simulink model "cirrusSR22T_v65"  (R2023a)
settings: Solver=ode45  StartTime=0.0  StopTime=360  FixedStep=0.001  MaxStep=0.1  RelTol=1e-3  EnableMultiTasking=on
values from neighbouring files (symbols this model uses):
  Aero_RP = [-1.145  0.0 -0.53]*[-1 0 0;0 1 0;0 0 -1]    [sr22t_data.m]
  aileron_limits = [-0.35 0.35]    [sr22t_data.m]
  Bw = 25.99*0.3048    (= 7.921752)    [sr22t_data.m]
  CD_alpha = [-1.57    1.500 ... (first row only)    [sr22t_data.m]
  CD_beta = [-1.57    1.230 ... (first row only)    [sr22t_data.m]
  CD_elev = 0.01    [sr22t_data.m]
  CD_ind = 0.007    [sr22t_data.m]
  CD_mach = [0, 0 ... (first row only)    [sr22t_data.m]
  Cl_ail = 0.1    [sr22t_data.m]
  CL_alpha = [-0.20 -0.750 ... (first row only)    [sr22t_data.m]
  Cl_beta = -0.1    [sr22t_data.m]
  CL_elev = 0.15    [sr22t_data.m]
  Cl_p = -0.4    [sr22t_data.m]
  CL_q = 3.9 * 0    (= 0)    [sr22t_data.m]
  Cl_r = 0.15    [sr22t_data.m]
  Cl_rudder = 0.01    [sr22t_data.m]
  Cm_alpha = -0.8    [sr22t_data.m]
  Cm_alpha_dot = -7    [sr22t_data.m]
  Cm_elev = [0.0, -1.100 ... (first row only)    [sr22t_data.m]
  Cm_q = -15    [sr22t_data.m]
  Cn_ail = -0.01    [sr22t_data.m]
  Cn_beta = 0.12    [sr22t_data.m]
  Cn_r = -0.15    [sr22t_data.m]
  Cn_rudder = -0.15    [sr22t_data.m]
  Cw = 5.58*0.3048    (= 1.700784)    [sr22t_data.m]
  CY_beta = -1    [sr22t_data.m]
  CY_p = [0.0000  -0.075 ... (first row only)    [sr22t_data.m]
  CY_r = [0.0000   0.214 ... (first row only)    [sr22t_data.m]
  CY_rudder = 0.187    [sr22t_data.m]
  Den = tf_linsys1(3,2).Denominator{1,1}    [controller_h_hold.m]
  elevator_limits = [-0.35 0.35]    [sr22t_data.m]
  He = tf_linsys1(3,2).Numerator{1,1}    [controller_h_hold.m]
  Href = 0.05 * x0(3)    [controller_h_hold.m]
  Ht = tf_linsys1(3,4).Numerator{1,1}    [controller_h_hold.m]
  isTrimming = 0    [sr22t_data.m]
  Jxx = 897*1.3558179    (= 1216.1686563)    [sr22t_data.m]
  Jxz = 0    [sr22t_data.m]
  Jyy = 20699*1.3558179    (= 28064.0747121)    [sr22t_data.m]
  Jzz = 19876*1.3558179    (= 26948.2365804)    [sr22t_data.m]
  Kp = 6    [controller_h_hold.m]
  kp = 0.005    [controller_h_hold.m]
  Kq = 3    [controller_h_hold.m]
  M = 2348*0.45359237    (= 1065.03488476)    [sr22t_data.m]
  Qe = tf_linsys1(8,2).Numerator{1,1}    [controller_h_hold.m]
  Qt = tf_linsys1(8,4).Numerator{1,1}    [controller_h_hold.m]
  Rcg = [-1.25 0.00 -0.54]*[-1 0 0;0 1 0;0 0 -1]    [sr22t_data.m]
  Rengine = [-3.6 0.0 -0.09045]*[-1 0 0;0 1 0;0 0 -1]    [sr22t_data.m]
  rudder_limits = [-0.35 0.35]    [sr22t_data.m]
  Sw = 144.92*0.09290304    (= 13.4635085568)    [sr22t_data.m]
  tau = 30    [controller_h_hold.m]
  Thetae = tf_linsys1(11,2).Numerator{1,1}    [controller_h_hold.m]
  Thetat = tf_linsys1(11,4).Numerator{1,1}    [controller_h_hold.m]
  thrust_limits = [0 1]    [sr22t_data.m]
  Ti = 17.5    [controller_h_hold.m]
  Tmax = M*10    (= 10650.3488476)    [sr22t_data.m]
  u0 = [op_trim1.Inputs(1,1).u, op_trim1.Inputs(2,1).u, op_trim1.Inputs(3,1).u, op_trim1.Inputs(4,1).u].'    [controller_h_hold.m]    (also in sr22t_data.m = [0, -0.013822, 0, 0.11837].')
  Ue = tf_linsys1(4,2).Numerator{1,1}    [controller_h_hold.m]
  Ut = tf_linsys1(4,4).Numerator{1,1}    [controller_h_hold.m]
  We = tf_linsys1(6,2).Numerator{1,1}    [controller_h_hold.m]
  Wt = tf_linsys1(6,4).Numerator{1,1}    [controller_h_hold.m]
  x0 = zeros(12,1)    [controller_h_hold.m]    (also in sr22t_data.m)
(part 2 of 2)

== system cirrusSR22T_v65/Cirrus SR22T/Aerodinamica/Forcas Aerodinamicas/Coef. Forca Lateral ==
  alpha : Inport
  beta : Inport  Port=2
  p : Inport  Port=3
  VT : Inport  Port=4
  r : Inport  Port=5
  rudder : Inport  Port=6
  CY_beta : Gain  Gain=CY_beta
  CY_p : Lookup  InputValues=CY_p(:,1);  Table=CY_p(:,2);  LookUpMeth=Interpolation-Use End Values
  CY_r : Lookup  InputValues=CY_r(:,1);  Table=CY_r(:,2);  LookUpMeth=Interpolation-Use End Values
  Constant2 : Constant  Value=Bw
  Gain : Gain  Gain=CY_rudder  SaturateOnIntegerOverflow=on  OutDataTypeStr=Inherit: Same as input  ParamDataTypeStr=Inherit: Same as input
  Gain1 : Gain  Gain=2  SaturateOnIntegerOverflow=on  OutDataTypeStr=Inherit: Same as input  ParamDataTypeStr=Inherit: Same as input
  Gain2 : Gain  Gain=0  SaturateOnIntegerOverflow=on  OutDataTypeStr=Inherit: Same as input  ParamDataTypeStr=Inherit: Same as input
  Gain3 : Gain  Gain=0  SaturateOnIntegerOverflow=on  OutDataTypeStr=Inherit: Same as input  ParamDataTypeStr=Inherit: Same as input
  Gain4 : Gain  Gain=0  SaturateOnIntegerOverflow=on  OutDataTypeStr=Inherit: Same as input  ParamDataTypeStr=Inherit: Same as input
  Product1 : Product  Inputs=3  SaturateOnIntegerOverflow=on  OutDataTypeStr=Inherit: Same as first input
  Product2 : Product  Inputs=3  SaturateOnIntegerOverflow=on  OutDataTypeStr=Inherit: Same as first input
  Product3 : Product  Inputs=*/  SaturateOnIntegerOverflow=on  OutDataTypeStr=Inherit: Same as first input
  Sum : Sum  Inputs=++++  SaturateOnIntegerOverflow=on
  C_Y : Outport
  wires:
  alpha/1 -> CY_p/1, CY_r/1
  beta/1 -> CY_beta/1
  Sum/1 -> C_Y/1
  CY_beta/1 -> Sum/1
  Product1/1 -> Sum/2
  p/1 -> Product1/2
  VT/1 -> Gain1/1
  Gain1/1 -> Product3/2
  Constant2/1 -> Product3/1
  Product3/1 -> Product1/3, Product2/1
  Product2/1 -> Sum/3
  CY_r/1 -> Gain2/1
  r/1 -> Product2/3
  Gain/1 -> Gain4/1
  rudder/1 -> Gain/1
  Gain2/1 -> Product2/2
  CY_p/1 -> Gain3/1
  Gain3/1 -> Product1/1
  Gain4/1 -> Sum/4

== system cirrusSR22T_v65/Cirrus SR22T/Aerodinamica/Forcas Aerodinamicas/Coef. sustentacao ==
  alpha : Inport
  elevator : Inport  Port=2
  VT : Inport  Port=3
  q : Inport  Port=4
  CL_alpha : Lookup  InputValues=CL_alpha(:,1);  Table=CL_alpha(:,2);  LookUpMeth=Interpolation-Use End Values
  Constant : Constant  Value=0
  Constant2 : Constant  Value=Cw
  Gain1 : Gain  Gain=2  SaturateOnIntegerOverflow=on  OutDataTypeStr=Inherit: Same as input  ParamDataTypeStr=Inherit: Same as input
  Gain2 : Gain  Gain=CL_q  SaturateOnIntegerOverflow=on  OutDataTypeStr=Inherit: Same as input  ParamDataTypeStr=Inherit: Same as input
  Gain3 : Gain  Gain=CL_elev  SaturateOnIntegerOverflow=on  OutDataTypeStr=Inherit: Same as input  ParamDataTypeStr=Inherit: Same as input
  Product2 : Product  SaturateOnIntegerOverflow=on  OutDataTypeStr=Inherit: Same as first input
  Product3 : Product  Inputs=*/  SaturateOnIntegerOverflow=on  OutDataTypeStr=Inherit: Same as first input
  Product4 : Product  SaturateOnIntegerOverflow=on  OutDataTypeStr=Inherit: Same as first input
  Sum1 : Sum  Inputs=++++  SaturateOnIntegerOverflow=on
  C_L : Outport
  wires:
  alpha/1 -> CL_alpha/1
  CL_alpha/1 -> Sum1/1
  Sum1/1 -> C_L/1
  Constant/1 -> Product2/1
  VT/1 -> Gain1/1
  Gain1/1 -> Product3/2
  Constant2/1 -> Product3/1
  Product2/1 -> Sum1/2
  Product3/1 -> Product2/2, Product4/2
  Gain2/1 -> Product4/1
  Product4/1 -> Sum1/3
  q/1 -> Gain2/1
  elevator/1 -> Gain3/1
  Gain3/1 -> Sum1/4

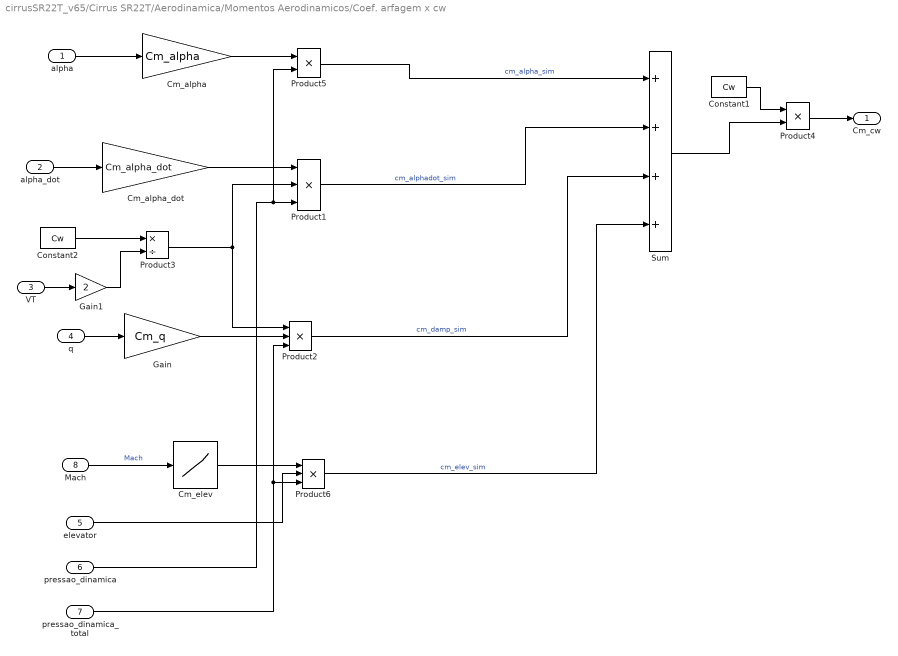
== system cirrusSR22T_v65/Cirrus SR22T/Aerodinamica/Momentos Aerodinamicos/Coef. arfagem x cw ==
  alpha : Inport
  alpha_dot : Inport  Port=2
  VT : Inport  Port=3
  q : Inport  Port=4
  elevator : Inport  Port=5
  pressao_dinamica : Inport  Port=6
  pressao_dinamica_total : Inport  Port=7
  Mach : Inport  Port=8
  Cm_alpha : Gain  Gain=Cm_alpha
  Cm_alpha_dot : Gain  Gain=Cm_alpha_dot
  Cm_elev : Lookup  InputValues=Cm_elev(:,1);  Table=Cm_elev(:,2);  LookUpMeth=Interpolation-Use End Values
  Constant1 : Constant  Value=Cw
  Constant2 : Constant  Value=Cw
  Gain : Gain  Gain=Cm_q  SaturateOnIntegerOverflow=on  OutDataTypeStr=Inherit: Same as input  ParamDataTypeStr=Inherit: Same as input
  Gain1 : Gain  Gain=2  SaturateOnIntegerOverflow=on  OutDataTypeStr=Inherit: Same as input  ParamDataTypeStr=Inherit: Same as input
  Product1 : Product  Inputs=***  SaturateOnIntegerOverflow=on  OutDataTypeStr=Inherit: Same as first input
  Product2 : Product  Inputs=***  SaturateOnIntegerOverflow=on  OutDataTypeStr=Inherit: Same as first input
  Product3 : Product  Inputs=*/  SaturateOnIntegerOverflow=on  OutDataTypeStr=Inherit: Same as first input
  Product4 : Product  Inputs=**  SaturateOnIntegerOverflow=on  OutDataTypeStr=Inherit: Same as first input
  Product5 : Product  Inputs=**  SaturateOnIntegerOverflow=on  OutDataTypeStr=Inherit: Same as first input
  Product6 : Product  Inputs=***  SaturateOnIntegerOverflow=on  OutDataTypeStr=Inherit: Same as first input
  Sum : Sum  Inputs=++++  SaturateOnIntegerOverflow=on
  Cm_cw : Outport
  wires:
  Constant1/1 -> Product4/1
  Sum/1 -> Product4/2
  Product4/1 -> Cm_cw/1
  VT/1 -> Gain1/1
  Gain1/1 -> Product3/2
  Constant2/1 -> Product3/1
  Cm_alpha_dot/1 -> Product1/1
  Product1/1 -> Sum/2  "cm_alphadot_sim"
  Product3/1 -> Product2/1, Product1/2
  q/1 -> Gain/1
  Gain/1 -> Product2/2
  Product2/1 -> Sum/3  "cm_damp_sim"
  elevator/1 -> Product6/2
  Mach/1 -> Cm_elev/1  "Mach"
  Cm_elev/1 -> Product6/1
  alpha_dot/1 -> Cm_alpha_dot/1
  alpha/1 -> Cm_alpha/1
  pressao_dinamica_total/1 -> Product2/3, Product6/3
  Product6/1 -> Sum/4  "cm_elev_sim"
  Cm_alpha/1 -> Product5/1
  Product5/1 -> Sum/1  "cm_alpha_sim"
  pressao_dinamica/1 -> Product5/2, Product1/3

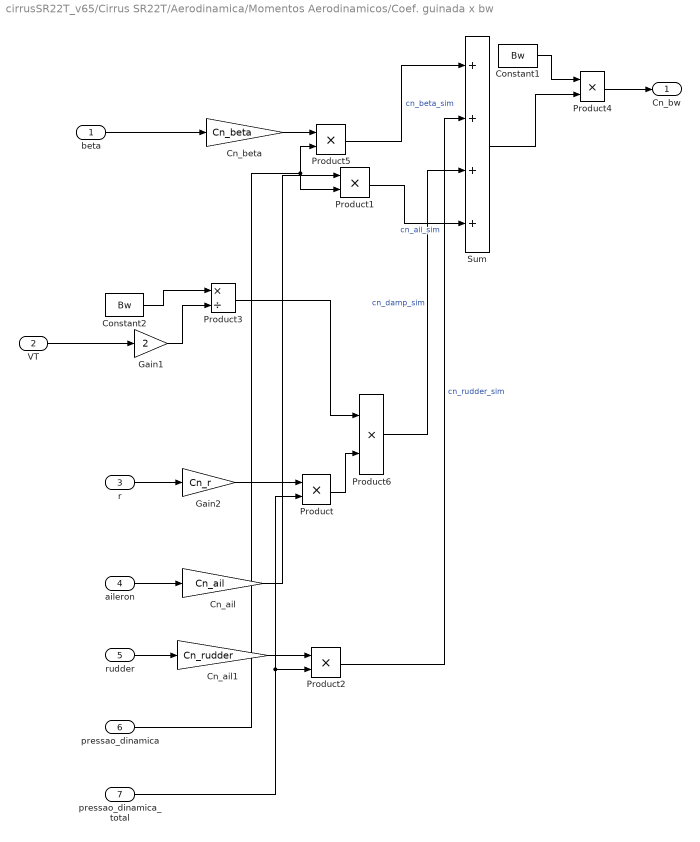
== system cirrusSR22T_v65/Cirrus SR22T/Aerodinamica/Momentos Aerodinamicos/Coef. guinada x bw ==
  beta : Inport
  VT : Inport  Port=2
  r : Inport  Port=3
  aileron : Inport  Port=4
  rudder : Inport  Port=5
  pressao_dinamica : Inport  Port=6
  pressao_dinamica_total : Inport  Port=7
  Cn_ail : Gain  Gain=Cn_ail  SaturateOnIntegerOverflow=on  OutDataTypeStr=Inherit: Same as input  ParamDataTypeStr=Inherit: Same as input
  Cn_ail1 : Gain  Gain=Cn_rudder  SaturateOnIntegerOverflow=on  OutDataTypeStr=Inherit: Same as input  ParamDataTypeStr=Inherit: Same as input
  Cn_beta : Gain  Gain=Cn_beta
  Constant1 : Constant  Value=Bw
  Constant2 : Constant  Value=Bw
  Gain1 : Gain  Gain=2  SaturateOnIntegerOverflow=on  OutDataTypeStr=Inherit: Same as input  ParamDataTypeStr=Inherit: Same as input
  Gain2 : Gain  Gain=Cn_r  SaturateOnIntegerOverflow=on  OutDataTypeStr=Inherit: Same as input  ParamDataTypeStr=Inherit: Same as input
  Product{,1..2,5} (4 alike) : Product
  Product3 : Product  Inputs=*/  SaturateOnIntegerOverflow=on  OutDataTypeStr=Inherit: Same as first input
  Product4 : Product  Inputs=**  SaturateOnIntegerOverflow=on  OutDataTypeStr=Inherit: Same as first input
  Product6 : Product  Inputs=**  SaturateOnIntegerOverflow=on  OutDataTypeStr=Inherit: Same as first input
  Sum : Sum  Inputs=++++  SaturateOnIntegerOverflow=on
  Cn_bw : Outport
  wires:
  Constant1/1 -> Product4/1
  Sum/1 -> Product4/2
  Product4/1 -> Cn_bw/1
  VT/1 -> Gain1/1
  Gain1/1 -> Product3/2
  Constant2/1 -> Product3/1
  beta/1 -> Cn_beta/1
  Product3/1 -> Product6/1
  r/1 -> Gain2/1
  Product6/1 -> Sum/3  "cn_damp_sim"
  aileron/1 -> Cn_ail/1
  rudder/1 -> Cn_ail1/1
  Gain2/1 -> Product/1
  Product/1 -> Product6/2
  pressao_dinamica_total/1 -> Product2/2, Product/2
  Cn_ail1/1 -> Product2/1
  Product2/1 -> Sum/2  "cn_rudder_sim"
  Cn_beta/1 -> Product5/1
  Product5/1 -> Sum/1  "cn_beta_sim"
  pressao_dinamica/1 -> Product1/2, Product5/2
  Product1/1 -> Sum/4  "cn_ail_sim"
  Cn_ail/1 -> Product1/1

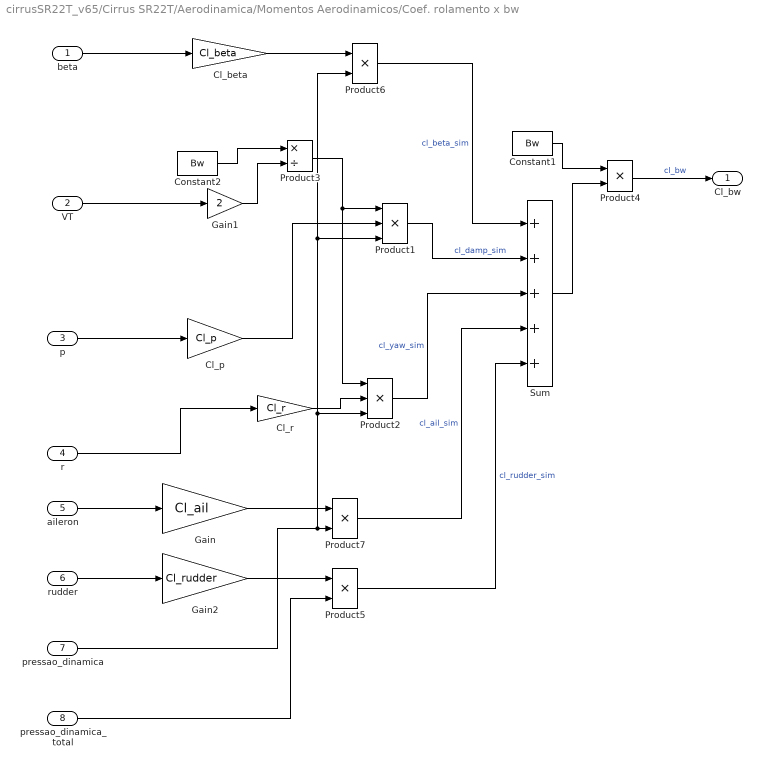
== system cirrusSR22T_v65/Cirrus SR22T/Aerodinamica/Momentos Aerodinamicos/Coef. rolamento x bw ==
  beta : Inport
  VT : Inport  Port=2
  p : Inport  Port=3
  r : Inport  Port=4
  aileron : Inport  Port=5
  rudder : Inport  Port=6
  pressao_dinamica : Inport  Port=7
  pressao_dinamica_total : Inport  Port=8
  Cl_beta : Gain  Gain=Cl_beta
  Cl_p : Gain  Gain=Cl_p
  Cl_r : Gain  Gain=Cl_r
  Constant1 : Constant  Value=Bw
  Constant2 : Constant  Value=Bw
  Gain : Gain  Gain=Cl_ail  SaturateOnIntegerOverflow=on  OutDataTypeStr=Inherit: Same as input  ParamDataTypeStr=Inherit: Same as input
  Gain1 : Gain  Gain=2  SaturateOnIntegerOverflow=on  OutDataTypeStr=Inherit: Same as input  ParamDataTypeStr=Inherit: Same as input
  Gain2 : Gain  Gain=Cl_rudder  SaturateOnIntegerOverflow=on  OutDataTypeStr=Inherit: Same as input  ParamDataTypeStr=Inherit: Same as input
  Product1 : Product  Inputs=3  SaturateOnIntegerOverflow=on  OutDataTypeStr=Inherit: Same as first input
  Product2 : Product  Inputs=3  SaturateOnIntegerOverflow=on  OutDataTypeStr=Inherit: Same as first input
  Product3 : Product  Inputs=*/  SaturateOnIntegerOverflow=on  OutDataTypeStr=Inherit: Same as first input
  Product4 : Product  Inputs=**  SaturateOnIntegerOverflow=on  OutDataTypeStr=Inherit: Same as first input
  Product5 : Product  SaturateOnIntegerOverflow=on  OutDataTypeStr=Inherit: Same as first input
  Product6 : Product  SaturateOnIntegerOverflow=on  OutDataTypeStr=Inherit: Same as first input
  Product7 : Product  SaturateOnIntegerOverflow=on  OutDataTypeStr=Inherit: Same as first input
  Sum : Sum  Inputs=+++++  SaturateOnIntegerOverflow=on
  Cl_bw : Outport
  wires:
  VT/1 -> Gain1/1
  Gain1/1 -> Product3/2
  Constant2/1 -> Product3/1
  Product3/1 -> Product2/1, Product1/1
  p/1 -> Cl_p/1
  r/1 -> Cl_r/1
  aileron/1 -> Gain/1
  rudder/1 -> Gain2/1
  Product1/1 -> Sum/2  "cl_damp_sim"
  Product2/1 -> Sum/3  "cl_yaw_sim"
  Constant1/1 -> Product4/1
  Sum/1 -> Product4/2
  Product4/1 -> Cl_bw/1  "cl_bw"
  beta/1 -> Cl_beta/1
  Cl_p/1 -> Product1/2
  Cl_r/1 -> Product2/2
  Gain2/1 -> Product5/1
  Product5/1 -> Sum/5  "cl_rudder_sim"
  pressao_dinamica_total/1 -> Product5/2
  pressao_dinamica/1 -> Product2/3, Product1/3, Product6/2, Product7/2
  Cl_beta/1 -> Product6/1
  Product6/1 -> Sum/1  "cl_beta_sim"
  Gain/1 -> Product7/1
  Product7/1 -> Sum/4  "cl_ail_sim"

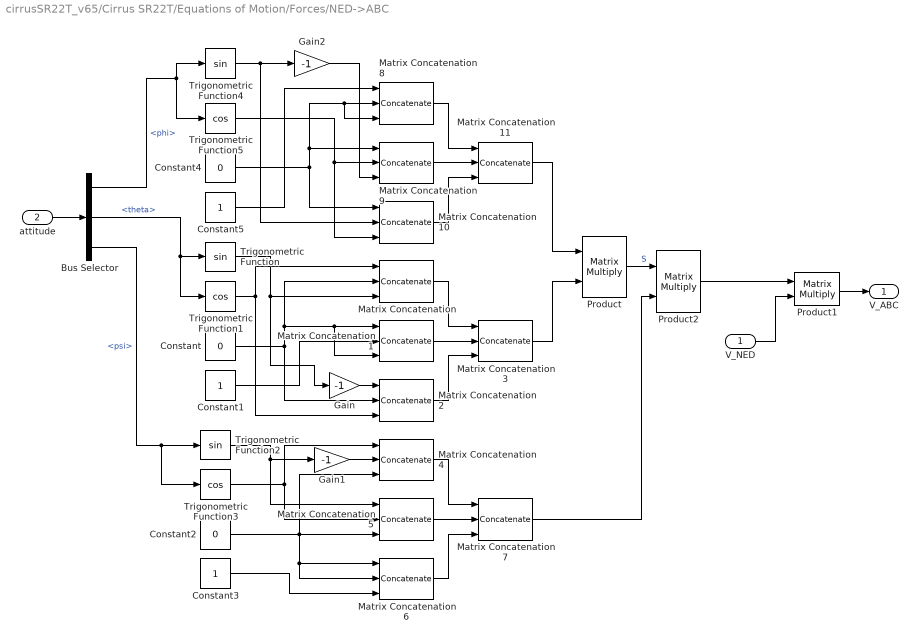
== system cirrusSR22T_v65/Cirrus SR22T/Equations of Motion/Forces/NED->ABC ==
  V_NED : Inport
  attitude : Inport  Port=2
  Bus Selector : BusSelector  OutputSignals=phi,theta,psi
  Constant : Constant  Value=0
  Constant1 : Constant
  Constant2 : Constant  Value=0
  Constant3 : Constant
  Constant4 : Constant  Value=0
  Constant5 : Constant
  Gain : Gain  Gain=-1  SaturateOnIntegerOverflow=on  OutDataTypeStr=Inherit: Same as input  ParamDataTypeStr=Inherit: Same as input
  Gain1 : Gain  Gain=-1  SaturateOnIntegerOverflow=on  OutDataTypeStr=Inherit: Same as input  ParamDataTypeStr=Inherit: Same as input
  Gain2 : Gain  Gain=-1  SaturateOnIntegerOverflow=on  OutDataTypeStr=Inherit: Same as input  ParamDataTypeStr=Inherit: Same as input
  Matrix Concatenation{,1..2,4..6,8..10} (9 alike) : Concatenate  NumInputs=3  Mode=Multidimensional array
  Matrix Concatenation11 : Concatenate  NumInputs=3  Mode=Multidimensional array  ConcatenateDimension=2
  Matrix Concatenation3 : Concatenate  NumInputs=3  Mode=Multidimensional array  ConcatenateDimension=2
  Matrix Concatenation7 : Concatenate  NumInputs=3  Mode=Multidimensional array  ConcatenateDimension=2
  Product : Product  Multiplication=Matrix(*)  SaturateOnIntegerOverflow=on  OutDataTypeStr=Inherit: Same as first input
  Product1 : Product  Multiplication=Matrix(*)  SaturateOnIntegerOverflow=on  OutDataTypeStr=Inherit: Same as first input
  Product2 : Product  Multiplication=Matrix(*)  SaturateOnIntegerOverflow=on  OutDataTypeStr=Inherit: Same as first input
  Trigonometric Function : Trigonometry
  Trigonometric Function1 : Trigonometry  Operator=cos
  Trigonometric Function2 : Trigonometry
  Trigonometric Function3 : Trigonometry  Operator=cos
  Trigonometric Function4 : Trigonometry
  Trigonometric Function5 : Trigonometry  Operator=cos
  V_ABC : Outport
  wires:
  Trigonometric Function1/1 -> Matrix Concatenation/1, Matrix Concatenation2/3
  Trigonometric Function/1 -> Matrix Concatenation/3, Gain/1
  Constant/1 -> Matrix Concatenation/2, Matrix Concatenation1/1, Matrix Concatenation1/3, Matrix Concatenation2/2
  Constant1/1 -> Matrix Concatenation1/2
  Matrix Concatenation/1 -> Matrix Concatenation3/1
  Matrix Concatenation1/1 -> Matrix Concatenation3/2
  Matrix Concatenation2/1 -> Matrix Concatenation3/3
  Matrix Concatenation4/1 -> Matrix Concatenation7/1
  Matrix Concatenation5/1 -> Matrix Concatenation7/2
  Matrix Concatenation6/1 -> Matrix Concatenation7/3
  Trigonometric Function3/1 -> Matrix Concatenation4/1, Matrix Concatenation5/2
  Trigonometric Function2/1 -> Gain1/1, Matrix Concatenation5/1
  Constant2/1 -> Matrix Concatenation4/3, Matrix Concatenation5/3, Matrix Concatenation6/1, Matrix Concatenation6/2
  Constant3/1 -> Matrix Concatenation6/3
  Product1/1 -> V_ABC/1
  attitude/1 -> Bus Selector/1
  Matrix Concatenation8/1 -> Matrix Concatenation11/1
  Matrix Concatenation9/1 -> Matrix Concatenation11/2
  Matrix Concatenation10/1 -> Matrix Concatenation11/3
  Bus Selector/1 -> Trigonometric Function4/1, Trigonometric Function5/1  "<phi>"
  Constant5/1 -> Matrix Concatenation8/1
  Constant4/1 -> Matrix Concatenation8/2, Matrix Concatenation8/3, Matrix Concatenation9/1, Matrix Concatenation10/1
  Trigonometric Function5/1 -> Matrix Concatenation9/2, Matrix Concatenation10/3
  Trigonometric Function4/1 -> Matrix Concatenation10/2, Gain2/1
  Bus Selector/2 -> Trigonometric Function/1, Trigonometric Function1/1  "<theta>"
  Bus Selector/3 -> Trigonometric Function2/1, Trigonometric Function3/1  "<psi>"
  Matrix Concatenation11/1 -> Product/1
  Matrix Concatenation3/1 -> Product/2
  V_NED/1 -> Product1/2
  Product/1 -> Product2/1  "S"
  Matrix Concatenation7/1 -> Product2/2
  Product2/1 -> Product1/1
  Gain2/1 -> Matrix Concatenation9/3
  Gain/1 -> Matrix Concatenation2/1
  Gain1/1 -> Matrix Concatenation4/2

== system cirrusSR22T_v65/Cirrus SR22T/Equations of Motion/Forces/Produto Vetorial ==
  V1 : Inport
  V2 : Inport  Port=2
  Mux : Mux  Inputs=2
  Mux1 : Mux  Inputs=3
  i : Fcn  Expr=u(2)*u(6)-u(3)*u(5)
  j : Fcn  Expr=-u(1)*u(6)+u(3)*u(4)
  k : Fcn  Expr=u(1)*u(5)-u(2)*u(4)
  V1 x V2 : Outport
  wires:
  V1/1 -> Mux/1
  V2/1 -> Mux/2
  Mux/1 -> i/1, j/1, k/1
  i/1 -> Mux1/1
  j/1 -> Mux1/2
  k/1 -> Mux1/3
  Mux1/1 -> V1 x V2/1

== system cirrusSR22T_v65/Cirrus SR22T/Equations of Motion/Forces/Produto Vetorial1 ==
  V1 : Inport
  V2 : Inport  Port=2
  Mux : Mux  Inputs=2
  Mux1 : Mux  Inputs=3
  i : Fcn  Expr=u(2)*u(6)-u(3)*u(5)
  j : Fcn  Expr=-u(1)*u(6)+u(3)*u(4)
  k : Fcn  Expr=u(1)*u(5)-u(2)*u(4)
  V1 x V2 : Outport
  wires:
  V1/1 -> Mux/1
  V2/1 -> Mux/2
  Mux/1 -> i/1, j/1, k/1
  i/1 -> Mux1/1
  j/1 -> Mux1/2
  k/1 -> Mux1/3
  Mux1/1 -> V1 x V2/1

== system cirrusSR22T_v65/Cirrus SR22T/Equations of Motion/Forces/Produto Vetorial2 ==
  V1 : Inport
  V2 : Inport  Port=2
  Mux : Mux  Inputs=2
  Mux1 : Mux  Inputs=3
  i : Fcn  Expr=u(2)*u(6)-u(3)*u(5)
  j : Fcn  Expr=-u(1)*u(6)+u(3)*u(4)
  k : Fcn  Expr=u(1)*u(5)-u(2)*u(4)
  V1 x V2 : Outport
  wires:
  V1/1 -> Mux/1
  V2/1 -> Mux/2
  Mux/1 -> i/1, j/1, k/1
  i/1 -> Mux1/1
  j/1 -> Mux1/2
  k/1 -> Mux1/3
  Mux1/1 -> V1 x V2/1

== system cirrusSR22T_v65/Cirrus SR22T/Equations of Motion/Forces/Produto Vetorial3 ==
  V1 : Inport
  V2 : Inport  Port=2
  Mux : Mux  Inputs=2
  Mux1 : Mux  Inputs=3
  i : Fcn  Expr=u(2)*u(6)-u(3)*u(5)
  j : Fcn  Expr=-u(1)*u(6)+u(3)*u(4)
  k : Fcn  Expr=u(1)*u(5)-u(2)*u(4)
  V1 x V2 : Outport
  wires:
  V1/1 -> Mux/1
  V2/1 -> Mux/2
  Mux/1 -> i/1, j/1, k/1
  i/1 -> Mux1/1
  j/1 -> Mux1/2
  k/1 -> Mux1/3
  Mux1/1 -> V1 x V2/1

== system cirrusSR22T_v65/Cirrus SR22T/Equations of Motion/Moments/Inertia ==
  Constant : Constant  Value=Jxx
  Constant1 : Constant  Value=Jyy
  Constant2 : Constant  Value=Jzz
  Constant3 : Constant  Value=-Jxz
  Constant4 : Constant  Value=0
  Matrix Concatenation10 : Concatenate  NumInputs=3  Mode=Multidimensional array
  Matrix Concatenation11 : Concatenate  NumInputs=3  Mode=Multidimensional array  ConcatenateDimension=2
  Matrix Concatenation8 : Concatenate  NumInputs=3  Mode=Multidimensional array
  Matrix Concatenation9 : Concatenate  NumInputs=3  Mode=Multidimensional array
  J : Outport
  wires:
  Matrix Concatenation8/1 -> Matrix Concatenation11/1
  Matrix Concatenation9/1 -> Matrix Concatenation11/2
  Matrix Concatenation10/1 -> Matrix Concatenation11/3
  Matrix Concatenation11/1 -> J/1
  Constant/1 -> Matrix Concatenation8/1
  Constant4/1 -> Matrix Concatenation8/2, Matrix Concatenation9/1, Matrix Concatenation9/3, Matrix Concatenation10/2
  Constant3/1 -> Matrix Concatenation8/3, Matrix Concatenation10/1
  Constant1/1 -> Matrix Concatenation9/2
  Constant2/1 -> Matrix Concatenation10/3

== system cirrusSR22T_v65/Cirrus SR22T/Equations of Motion/Moments/Inverse Inertia Matrix ==
  Constant : Constant  Value=Jzz
  Constant1 : Constant  Value=1/Jyy
  Constant2 : Constant  Value=Jxx
  Constant3 : Constant  Value=Jxz
  Constant4 : Constant  Value=0
  Constant5 : Constant  Value=Jxx*Jzz-Jxz^2
  Matrix Concatenation10 : Concatenate  NumInputs=3  Mode=Multidimensional array
  Matrix Concatenation11 : Concatenate  NumInputs=3  Mode=Multidimensional array  ConcatenateDimension=2
  Matrix Concatenation8 : Concatenate  NumInputs=3  Mode=Multidimensional array
  Matrix Concatenation9 : Concatenate  NumInputs=3  Mode=Multidimensional array
  Product : Product  Inputs=*/  SaturateOnIntegerOverflow=on  OutDataTypeStr=Inherit: Same as first input
  Product1 : Product  SaturateOnIntegerOverflow=on  OutDataTypeStr=Inherit: Same as first input
  inv J : Outport
  wires:
  Matrix Concatenation8/1 -> Matrix Concatenation11/1
  Matrix Concatenation9/1 -> Matrix Concatenation11/2
  Matrix Concatenation10/1 -> Matrix Concatenation11/3
  Constant/1 -> Matrix Concatenation8/1
  Constant4/1 -> Matrix Concatenation8/2, Matrix Concatenation9/1, Matrix Concatenation9/3, Matrix Concatenation10/2
  Constant3/1 -> Matrix Concatenation8/3, Matrix Concatenation10/1
  Constant2/1 -> Matrix Concatenation10/3
  Matrix Concatenation11/1 -> Product/1
  Product/1 -> inv J/1
  Constant5/1 -> Product/2, Product1/2
  Constant1/1 -> Product1/1
  Product1/1 -> Matrix Concatenation9/2

== system cirrusSR22T_v65/Cirrus SR22T/Equations of Motion/Moments/Produto Vetorial1 ==
  V1 : Inport
  V2 : Inport  Port=2
  Mux : Mux  Inputs=2
  Mux1 : Mux  Inputs=3
  i : Fcn  Expr=u(2)*u(6)-u(3)*u(5)
  j : Fcn  Expr=-u(1)*u(6)+u(3)*u(4)
  k : Fcn  Expr=u(1)*u(5)-u(2)*u(4)
  V1 x V2 : Outport
  wires:
  V1/1 -> Mux/1
  V2/1 -> Mux/2
  Mux/1 -> i/1, j/1, k/1
  i/1 -> Mux1/1
  j/1 -> Mux1/2
  k/1 -> Mux1/3
  Mux1/1 -> V1 x V2/1

== system cirrusSR22T_v65/Cirrus SR22T/Equations of Motion/Moments/Produto Vetorial2 ==
  V1 : Inport
  V2 : Inport  Port=2
  Mux : Mux  Inputs=2
  Mux1 : Mux  Inputs=3
  i : Fcn  Expr=u(2)*u(6)-u(3)*u(5)
  j : Fcn  Expr=-u(1)*u(6)+u(3)*u(4)
  k : Fcn  Expr=u(1)*u(5)-u(2)*u(4)
  V1 x V2 : Outport
  wires:
  V1/1 -> Mux/1
  V2/1 -> Mux/2
  Mux/1 -> i/1, j/1, k/1
  i/1 -> Mux1/1
  j/1 -> Mux1/2
  k/1 -> Mux1/3
  Mux1/1 -> V1 x V2/1

== system cirrusSR22T_v65/Cirrus SR22T/Equations of Motion/Moments/Produto Vetorial3 ==
  V1 : Inport
  V2 : Inport  Port=2
  Mux : Mux  Inputs=2
  Mux1 : Mux  Inputs=3
  i : Fcn  Expr=u(2)*u(6)-u(3)*u(5)
  j : Fcn  Expr=-u(1)*u(6)+u(3)*u(4)
  k : Fcn  Expr=u(1)*u(5)-u(2)*u(4)
  V1 x V2 : Outport
  wires:
  V1/1 -> Mux/1
  V2/1 -> Mux/2
  Mux/1 -> i/1, j/1, k/1
  i/1 -> Mux1/1
  j/1 -> Mux1/2
  k/1 -> Mux1/3
  Mux1/1 -> V1 x V2/1

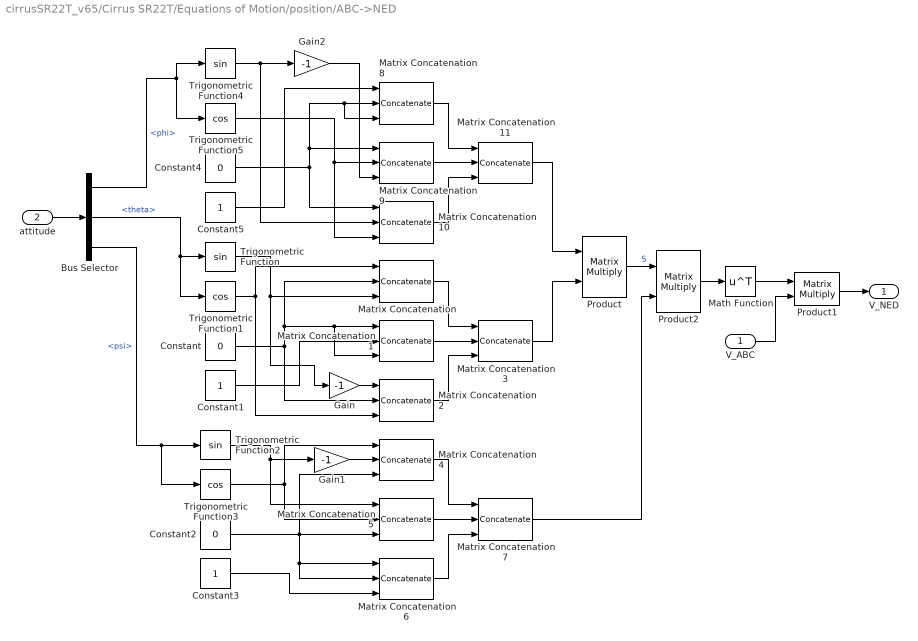
== system cirrusSR22T_v65/Cirrus SR22T/Equations of Motion/position/ABC->NED ==
  V_ABC : Inport
  attitude : Inport  Port=2
  Bus Selector : BusSelector  OutputSignals=phi,theta,psi
  Constant : Constant  Value=0
  Constant1 : Constant
  Constant2 : Constant  Value=0
  Constant3 : Constant
  Constant4 : Constant  Value=0
  Constant5 : Constant
  Gain : Gain  Gain=-1  SaturateOnIntegerOverflow=on  OutDataTypeStr=Inherit: Same as input  ParamDataTypeStr=Inherit: Same as input
  Gain1 : Gain  Gain=-1  SaturateOnIntegerOverflow=on  OutDataTypeStr=Inherit: Same as input  ParamDataTypeStr=Inherit: Same as input
  Gain2 : Gain  Gain=-1  SaturateOnIntegerOverflow=on  OutDataTypeStr=Inherit: Same as input  ParamDataTypeStr=Inherit: Same as input
  Math Function : Math  Operator=transpose  SignedPower=on
  Matrix Concatenation{,1..2,4..6,8..10} (9 alike) : Concatenate  NumInputs=3  Mode=Multidimensional array
  Matrix Concatenation11 : Concatenate  NumInputs=3  Mode=Multidimensional array  ConcatenateDimension=2
  Matrix Concatenation3 : Concatenate  NumInputs=3  Mode=Multidimensional array  ConcatenateDimension=2
  Matrix Concatenation7 : Concatenate  NumInputs=3  Mode=Multidimensional array  ConcatenateDimension=2
  Product : Product  Multiplication=Matrix(*)  SaturateOnIntegerOverflow=on  OutDataTypeStr=Inherit: Same as first input
  Product1 : Product  Multiplication=Matrix(*)  SaturateOnIntegerOverflow=on  OutDataTypeStr=Inherit: Same as first input
  Product2 : Product  Multiplication=Matrix(*)  SaturateOnIntegerOverflow=on  OutDataTypeStr=Inherit: Same as first input
  Trigonometric Function : Trigonometry
  Trigonometric Function1 : Trigonometry  Operator=cos
  Trigonometric Function2 : Trigonometry
  Trigonometric Function3 : Trigonometry  Operator=cos
  Trigonometric Function4 : Trigonometry
  Trigonometric Function5 : Trigonometry  Operator=cos
  V_NED : Outport
  wires:
  Trigonometric Function1/1 -> Matrix Concatenation/1, Matrix Concatenation2/3
  Trigonometric Function/1 -> Matrix Concatenation/3, Gain/1
  Constant/1 -> Matrix Concatenation/2, Matrix Concatenation1/1, Matrix Concatenation1/3, Matrix Concatenation2/2
  Constant1/1 -> Matrix Concatenation1/2
  Matrix Concatenation/1 -> Matrix Concatenation3/1
  Matrix Concatenation1/1 -> Matrix Concatenation3/2
  Matrix Concatenation2/1 -> Matrix Concatenation3/3
  Matrix Concatenation4/1 -> Matrix Concatenation7/1
  Matrix Concatenation5/1 -> Matrix Concatenation7/2
  Matrix Concatenation6/1 -> Matrix Concatenation7/3
  Trigonometric Function3/1 -> Matrix Concatenation4/1, Matrix Concatenation5/2
  Trigonometric Function2/1 -> Gain1/1, Matrix Concatenation5/1
  Constant2/1 -> Matrix Concatenation4/3, Matrix Concatenation5/3, Matrix Concatenation6/1, Matrix Concatenation6/2
  Constant3/1 -> Matrix Concatenation6/3
  Product1/1 -> V_NED/1
  attitude/1 -> Bus Selector/1
  Matrix Concatenation8/1 -> Matrix Concatenation11/1
  Matrix Concatenation9/1 -> Matrix Concatenation11/2
  Matrix Concatenation10/1 -> Matrix Concatenation11/3
  Bus Selector/1 -> Trigonometric Function4/1, Trigonometric Function5/1  "<phi>"
  Constant5/1 -> Matrix Concatenation8/1
  Constant4/1 -> Matrix Concatenation8/2, Matrix Concatenation8/3, Matrix Concatenation9/1, Matrix Concatenation10/1
  Trigonometric Function5/1 -> Matrix Concatenation9/2, Matrix Concatenation10/3
  Trigonometric Function4/1 -> Matrix Concatenation10/2, Gain2/1
  Bus Selector/2 -> Trigonometric Function/1, Trigonometric Function1/1  "<theta>"
  Bus Selector/3 -> Trigonometric Function2/1, Trigonometric Function3/1  "<psi>"
  Matrix Concatenation11/1 -> Product/1
  Matrix Concatenation3/1 -> Product/2
  V_ABC/1 -> Product1/2
  Product/1 -> Product2/1  "S"
  Matrix Concatenation7/1 -> Product2/2
  Gain2/1 -> Matrix Concatenation9/3
  Gain/1 -> Matrix Concatenation2/1
  Gain1/1 -> Matrix Concatenation4/2
  Product2/1 -> Math Function/1
  Math Function/1 -> Product1/1
